simulink model "Assignment2_3"  (R2021a)
settings: Solver=VariableStepAuto  StartTime=0.0  StopTime=10  RelTol=1e-3
settings Model: Creator=mstra  LastModifiedBy=mstra
settings SolverCC: AlgebraicLoopSolver=TrustRegion
settings DebuggingCC: SFMachineParentedDataDiag=warning

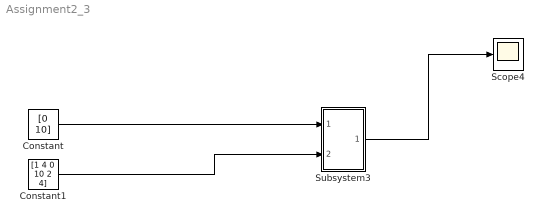
== system Assignment2_3 ==
  Constant : Constant  Value=[0 10]
  Constant1 : Constant  Value=[1 4 0 10 2 4]
  Scope4 : Scope
  Subsystem3 : Subsystem
  wires:
  Constant/1 -> Subsystem3/1(In1)
  Constant1/1 -> Subsystem3/2(In2)
  Subsystem3/1(Out1) -> Scope4/1

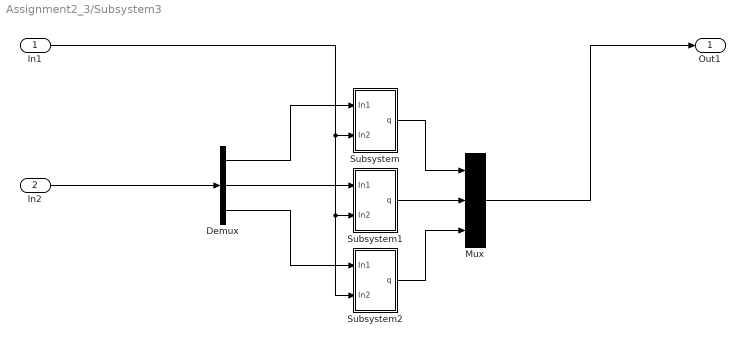
== system Assignment2_3/Subsystem3 ==
  In1 : Inport
  In2 : Inport  Port=2
  Demux : Demux  Outputs=3
  Mux : Mux  Inputs=3
  Subsystem : Subsystem
  Subsystem1 : Subsystem
  Subsystem2 : Subsystem
  Out1 : Outport
  wires:
  Demux/3 -> Subsystem2/1(In1)
  Subsystem2/1(q) -> Mux/3
  In1/1 -> Subsystem1/2(In2), Subsystem2/2(In2), Subsystem/2(In2)
  Subsystem/1(q) -> Mux/1
  Demux/2 -> Subsystem1/1(In1)
  Demux/1 -> Subsystem/1(In1)
  Subsystem1/1(q) -> Mux/2
  In2/1 -> Demux/1
  Mux/1 -> Out1/1

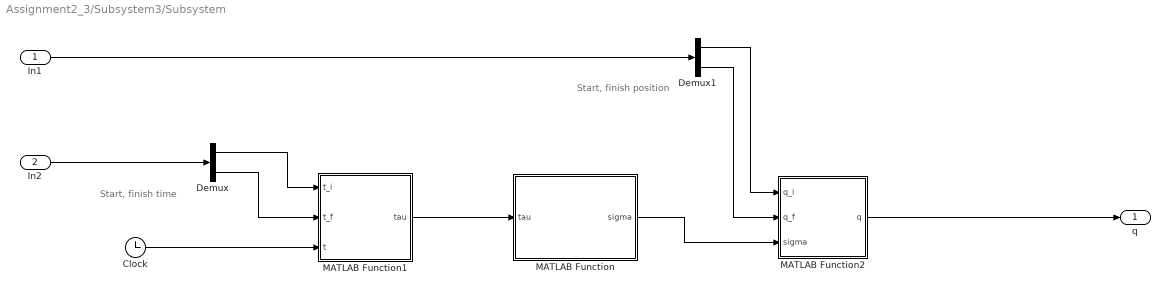
== system Assignment2_3/Subsystem3/Subsystem ==
  note: Start, finish position
  note: Start, finish time
  In1 : Inport
  In2 : Inport  Port=2
  Clock : Clock
  Demux : Demux  Outputs=2
  Demux1 : Demux  Outputs=2
  MATLAB Function : MATLAB Function  TreatAsAtomicUnit=on
  MATLAB Function1 : MATLAB Function  TreatAsAtomicUnit=on
  MATLAB Function2 : MATLAB Function  TreatAsAtomicUnit=on
  q : Outport
  wires:
  MATLAB Function1/1(tau) -> MATLAB Function/1(tau)
  Demux1/2 -> MATLAB Function2/2(q_f)
  Demux/1 -> MATLAB Function1/1(t_i)
  Clock/1 -> MATLAB Function1/3(t)
  Demux/2 -> MATLAB Function1/2(t_f)
  MATLAB Function/1(sigma) -> MATLAB Function2/3(sigma)
  MATLAB Function2/1(q) -> q/1
  In2/1 -> Demux/1
  Demux1/1 -> MATLAB Function2/1(q_i)
  In1/1 -> Demux1/1

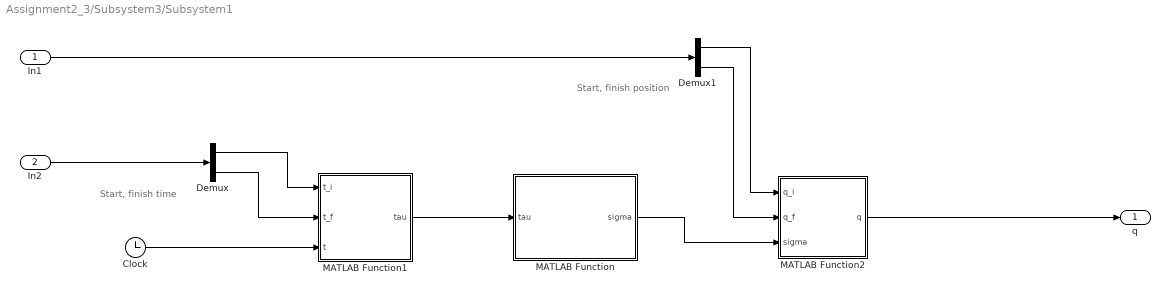
== system Assignment2_3/Subsystem3/Subsystem1 ==
  note: Start, finish position
  note: Start, finish time
  In1 : Inport
  In2 : Inport  Port=2
  Clock : Clock
  Demux : Demux  Outputs=2
  Demux1 : Demux  Outputs=2
  MATLAB Function : MATLAB Function  TreatAsAtomicUnit=on
  MATLAB Function1 : MATLAB Function  TreatAsAtomicUnit=on
  MATLAB Function2 : MATLAB Function  TreatAsAtomicUnit=on
  q : Outport
  wires:
  MATLAB Function1/1(tau) -> MATLAB Function/1(tau)
  Demux1/2 -> MATLAB Function2/2(q_f)
  Demux/1 -> MATLAB Function1/1(t_i)
  Clock/1 -> MATLAB Function1/3(t)
  Demux/2 -> MATLAB Function1/2(t_f)
  MATLAB Function/1(sigma) -> MATLAB Function2/3(sigma)
  MATLAB Function2/1(q) -> q/1
  In2/1 -> Demux/1
  Demux1/1 -> MATLAB Function2/1(q_i)
  In1/1 -> Demux1/1

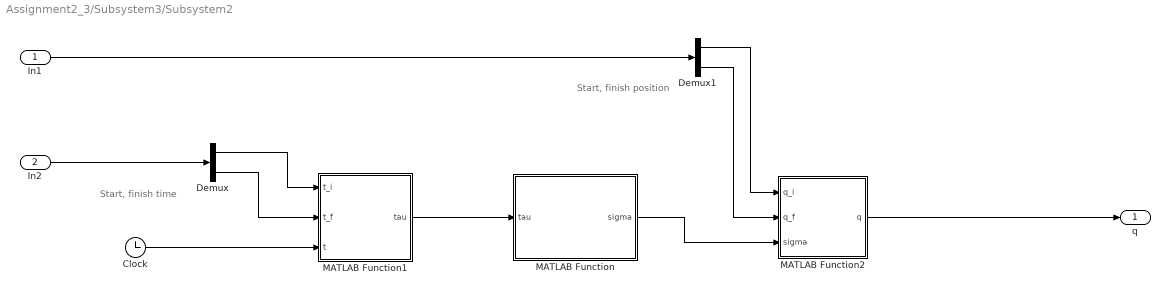
== system Assignment2_3/Subsystem3/Subsystem2 ==
  note: Start, finish position
  note: Start, finish time
  In1 : Inport
  In2 : Inport  Port=2
  Clock : Clock
  Demux : Demux  Outputs=2
  Demux1 : Demux  Outputs=2
  MATLAB Function : MATLAB Function  TreatAsAtomicUnit=on
  MATLAB Function1 : MATLAB Function  TreatAsAtomicUnit=on
  MATLAB Function2 : MATLAB Function  TreatAsAtomicUnit=on
  q : Outport
  wires:
  MATLAB Function1/1(tau) -> MATLAB Function/1(tau)
  Demux1/2 -> MATLAB Function2/2(q_f)
  Demux/1 -> MATLAB Function1/1(t_i)
  Clock/1 -> MATLAB Function1/3(t)
  Demux/2 -> MATLAB Function1/2(t_f)
  MATLAB Function/1(sigma) -> MATLAB Function2/3(sigma)
  MATLAB Function2/1(q) -> q/1
  In2/1 -> Demux/1
  Demux1/1 -> MATLAB Function2/1(q_i)
  In1/1 -> Demux1/1

== matlab function Assignment2_3/Subsystem3/Subsystem/MATLAB Function1 ==
  data: t_i input; tau output; t_f input; t input
function tau = t2tau(t_i,t_f,t)
% Compute the value of tau. 
% INPUT: 
% -	t_i: initial time 
% -	t_f: final time 
% - t: symbolic time variable
% OUTPUT:
% - tau 
%

T = t_f - t_i;
tau = (t - t_i)/T;

== matlab function Assignment2_3/Subsystem3/Subsystem/MATLAB Function ==
  data: sigma output; tau input
function sigma  = sim_poly_trajD5(tau)
% Compute sigma
% INPUT: 
% - tau 
% OUTPUT: 
% - sigma 

sigma = 10*tau^3 - 15*tau^4 + 6*tau^5;

end

== matlab function Assignment2_3/Subsystem3/Subsystem/MATLAB Function2 ==
  data: q_i input; q output; q_f input; sigma input
function q = fcn(q_i,q_f,sigma)
% compute position at time t
% INPUT: 
% -	q_i: initial value (i.e., value at t_i) 
% -	q_f: final value (i.e., value at time t_f) 
% - sigma
% OUTPUT:
% - q: position at time t

h = q_f - q_i;
q = q_i + h * sigma;

== matlab function Assignment2_3/Subsystem3/Subsystem1/MATLAB Function ==
  data: sigma output; tau input
function sigma  = sim_poly_trajD5(tau)
% Compute sigma
% INPUT: 
% - tau 
% OUTPUT: 
% - sigma 

sigma = 10*tau^3 - 15*tau^4 + 6*tau^5;

end

== matlab function Assignment2_3/Subsystem3/Subsystem1/MATLAB Function1 ==
  data: t_i input; tau output; t_f input; t input
function tau = t2tau(t_i,t_f,t)
% Compute the value of tau. 
% INPUT: 
% -	t_i: initial time 
% -	t_f: final time 
% - t: symbolic time variable
% OUTPUT:
% - tau 
%

T = t_f - t_i;
tau = (t - t_i)/T;

== matlab function Assignment2_3/Subsystem3/Subsystem1/MATLAB Function2 ==
  data: q_i input; q output; q_f input; sigma input
function q = fcn(q_i,q_f,sigma)
% compute position at time t
% INPUT: 
% -	q_i: initial value (i.e., value at t_i) 
% -	q_f: final value (i.e., value at time t_f) 
% - sigma
% OUTPUT:
% - q: position at time t

h = q_f - q_i;
q = q_i + h * sigma;

== matlab function Assignment2_3/Subsystem3/Subsystem2/MATLAB Function ==
  data: sigma output; tau input
function sigma  = sim_poly_trajD5(tau)
% Compute sigma
% INPUT: 
% - tau 
% OUTPUT: 
% - sigma 

sigma = 10*tau^3 - 15*tau^4 + 6*tau^5;

end

== matlab function Assignment2_3/Subsystem3/Subsystem2/MATLAB Function1 ==
  data: t_i input; tau output; t_f input; t input
function tau = t2tau(t_i,t_f,t)
% Compute the value of tau. 
% INPUT: 
% -	t_i: initial time 
% -	t_f: final time 
% - t: symbolic time variable
% OUTPUT:
% - tau 
%

T = t_f - t_i;
tau = (t - t_i)/T;

== matlab function Assignment2_3/Subsystem3/Subsystem2/MATLAB Function2 ==
  data: q_i input; q output; q_f input; sigma input
function q = fcn(q_i,q_f,sigma)
% compute position at time t
% INPUT: 
% -	q_i: initial value (i.e., value at t_i) 
% -	q_f: final value (i.e., value at time t_f) 
% - sigma
% OUTPUT:
% - q: position at time t

h = q_f - q_i;
q = q_i + h * sigma;
